simulink model "LQR_Lineal_vs_NoLineal"  (R2025b)
settings: Solver=ode45  StartTime=0.0  StopTime=10  RelTol=1e-3
values from neighbouring files (symbols this model uses):
  A_num = zeros(6,6)    [segway_sim_lazo_abierto.m]
  K = place(A, B, polos_deseados)    [segway_controlador.m]
undefined symbols (not defined in the file or in its folder): B_aug, C_num, D_aug
settings Model: Creator=crist  LastModifiedBy=crist

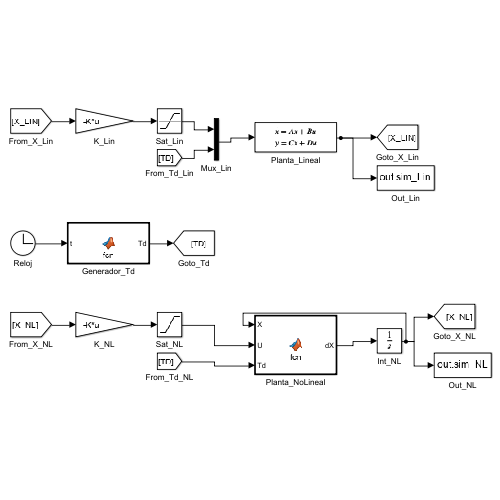
[thumbnail: Simulink's stored preview of the top-level diagram]
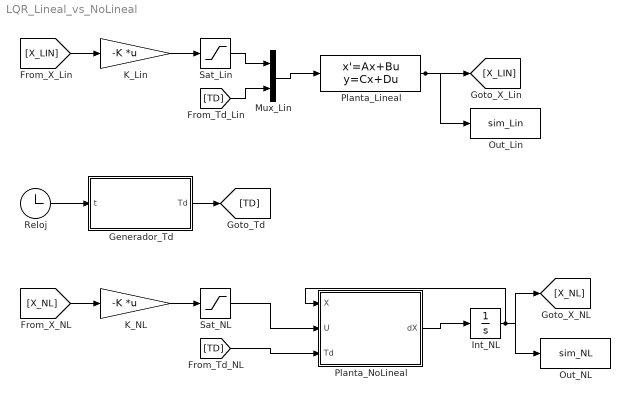
== system LQR_Lineal_vs_NoLineal ==
  Generador_Td : MATLAB Function  TreatAsAtomicUnit=on
  Int_NL : Integrator  InitialCondition=zeros(6,1)
  K_Lin : Gain  Gain=-K  Multiplication=Matrix(K*u)
  K_NL : Gain  Gain=-K  Multiplication=Matrix(K*u)
  Mux_Lin : Mux  Inputs=2
  Out_Lin : ToWorkspace  VariableName=sim_Lin  SampleTime=-1
  Out_NL : ToWorkspace  VariableName=sim_NL  SampleTime=-1
  Planta_Lineal : StateSpace  A=A_num  B=B_aug  C=C_num  D=D_aug  InitialCondition=zeros(6,1)
  Planta_NoLineal : MATLAB Function  TreatAsAtomicUnit=on
  Reloj : Clock
  Sat_Lin : Saturate  UpperLimit=24  LowerLimit=-24
  Sat_NL : Saturate  UpperLimit=24  LowerLimit=-24
  wires:
  Reloj/1 -> Generador_Td/1(t)
  Generador_Td/1(Td) -> [TD]
  [X_LIN] -> K_Lin/1
  K_Lin/1 -> Sat_Lin/1
  Sat_Lin/1 -> Mux_Lin/1
  [TD] -> Mux_Lin/2
  Mux_Lin/1 -> Planta_Lineal/1
  Planta_Lineal/1 -> [X_LIN], Out_Lin/1
  [X_NL] -> K_NL/1
  K_NL/1 -> Sat_NL/1
  Int_NL/1 -> Planta_NoLineal/1(X), [X_NL], Out_NL/1
  Sat_NL/1 -> Planta_NoLineal/2(U)
  [TD] -> Planta_NoLineal/3(Td)
  Planta_NoLineal/1(dX) -> Int_NL/1

== matlab function LQR_Lineal_vs_NoLineal/Generador_Td ==
  data: t input; Td output
function Td = fcn(t)
    % Perturbación de 15 Nm entre 2s y 6s
    if t >= 2 && t <= 6
        Td = 15;
    else
        Td = 0;
    end
end

== matlab function LQR_Lineal_vs_NoLineal/Planta_NoLineal ==
  data: X input; dX output; U input; Td input
function dX = fcn(X, U, Td)
    % Parámetros Físicos
    M = 80; m = 2; r = 0.20; d = 0.60; l = 0.90; g = 9.81;
    Icy = 10; Icz = 12; Icx = 12; Iw = 0.08; Iwz = 0.04;
    alpha_m = 2.0; beta_m = 1.5;
    % Desglose de Entradas
    theta = X(1); dtheta = X(2); dx = X(4); dalpha = X(6);
    VR = U(1); VL = U(2);
    % Dinámica Física No Lineal
    omega_Rw = dx/r + d/(2*r)*dalpha; omega_Lw = dx/r - d/(2*r)*dalpha;
    tau_R = alpha_m*VR - beta_m*(omega_Rw - dtheta);
    tau_L = alpha_m*VL - beta_m*(omega_Lw - dtheta);
    M11 = Icy + M*l^2; M12 = M*l*cos(theta); M22 = M + 2*m + 2*Iw/r^2;
    detM = M11*M22 - M12^2;
    F1 = M*g*l*sin(theta) - (tau_R + tau_L) + Td;
    F2 = M*l*dtheta^2*sin(theta) + (tau_R + tau_L)/r;
    ddtheta = ( M22*F1 - M12*F2) / detM;
    ddx     = (-M12*F1 + M11*F2) / detM;
    M33 = Icz + 2*m*(d/2)^2 + 2*Iw*(d/(2*r)^2) + Iwz;
    ddalpha = (d*(tau_R - tau_L)/(2*r)) / M33;
    dX = [dtheta; ddtheta; dx; ddx; dalpha; ddalpha];
end
